simulink model "Eg1"  (R2014a)
settings: Solver=ode45  StartTime=0.0  StopTime=10.0  RelTol=1e-3
settings Model: Creator=Administrator  LastModifiedBy=Administrator

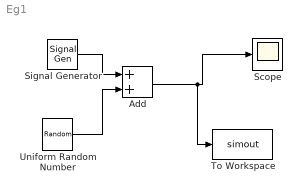
== system Eg1 ==
  Add : Sum
  Scope : Scope
  Signal Generator : SignalGenerator  Amplitude=2  Frequency=0.5
  To Workspace : ToWorkspace  VariableName=simout  SaveFormat=Timeseries  SampleTime=-1
  Uniform Random Number : UniformRandomNumber  SampleTime=0.1
  wires:
  Signal Generator/1 -> Add/1
  Uniform Random Number/1 -> Add/2
  Add/1 -> To Workspace/1, Scope/1
